simulink model "hcc_sm_v6_circuit2"  (R2024b)
settings: Solver=VariableStepAuto  StartTime=0.0  StopTime=0.2  RelTol=1e-3
libraries: spsSeriesRLCBranchLib x530, spsGtoLib x144, spsDiodeLib x78, spsVoltageMeasurementLib x6, spsGroundLib x2, spsDCVoltageSourceLib x1, spsNonlinearResistorLib x1, spsThreePhaseTransformerTwoWindingsLib x1, spsThreePhaseSourceLib x1, spspowerguiLib x1
(part 2 of 3)

== system hcc_sm_v6_circuit2/Bridge4/Segment3 ==
  gate : Inport
  C{101..106} (6 alike) : spsSeriesRLCBranchLib/Series RLC Branch  LConnTagsString=__new0  RConnTagsString=__new0  BranchType=C  Resistance=350  Inductance=107.42e-03  SetiL0=off  InitialCurrent=0  Capacitance=2.2*1e-6  Setx0=off  InitialVoltage=0  Measurements=None
  Gto{1..6} (6 alike) : spsGtoLib/Gto  Ron=0.226e-6  Lon=0  Vf=1.2  Tf=10e-6  Tt=20e-6  IC=0  Rs=161.25e3  Cs=0  Measurements=off
  R{101..106} (6 alike) : spsSeriesRLCBranchLib/Series RLC Branch  LConnTagsString=__new0  RConnTagsString=__new0  BranchType=R  Resistance=36  Inductance=107.42e-03  SetiL0=off  InitialCurrent=0  Capacitance=2.62e-06  Setx0=off  InitialVoltage=0  Measurements=None
  R{201..206} (6 alike) : spsSeriesRLCBranchLib/Series RLC Branch  LConnTagsString=__new0  RConnTagsString=__new0  BranchType=R  Resistance=88  Inductance=107.42e-03  SetiL0=off  InitialCurrent=0  Capacitance=2.62e-06  Setx0=off  InitialVoltage=0  Measurements=None
  R301_replace : spsDiodeLib/Diode  Ron=0.2624  Lon=0  Vf=11825.10104  IC=0  UseSnubber=0  Rs=1e6  Cs=0  Measurements=on
  R301_replace1 : spsDiodeLib/Diode  Ron=0.2624  Lon=0  Vf=11825.10104  IC=0  UseSnubber=0  Rs=1e6  Cs=0  Measurements=on
  R301_replace2 : spsDiodeLib/Diode  Ron=0.2624  Lon=0  Vf=11825.10104  IC=0  UseSnubber=0  Rs=1e6  Cs=0  Measurements=on
  SaturableReactor : Subsystem
  top : PMIOPort  Side=Left
  bottom : PMIOPort  Port=2  Side=Right
  wires:
  gate/1 -> Gto1/1, Gto2/1, Gto5/1, Gto6/1, Gto4/1, Gto3/1
  connections:
  R106/RConn1 -- C106/LConn1
  R105/RConn1 -- C105/LConn1
  R104/RConn1 -- C104/LConn1
  R103/RConn1 -- C103/LConn1
  C102/LConn1 -- R102/RConn1
  C101/LConn1 -- R101/RConn1
  SaturableReactor/LConn1 -- top/RConn1
  bottom/RConn1 -- R206/RConn1 -- Gto6/RConn1 -- C106/RConn1 -- R301_replace2/RConn1
  R301_replace2/LConn1 -- R301_replace1/RConn1 -- R204/RConn1 -- R205/LConn1 -- Gto4/RConn1 -- Gto5/LConn1 -- C104/RConn1 -- R105/LConn1
  R301_replace1/LConn1 -- R301_replace/RConn1 -- R202/RConn1 -- R103/LConn1 -- Gto2/RConn1 -- Gto3/LConn1 -- C102/RConn1 -- R203/LConn1
  R206/LConn1 -- Gto5/RConn1 -- Gto6/LConn1 -- R106/LConn1 -- C105/RConn1 -- R205/RConn1
  R301_replace/LConn1 -- R101/LConn1 -- SaturableReactor/RConn1 -- Gto1/LConn1 -- R201/LConn1
  R104/LConn1 -- Gto3/RConn1 -- Gto4/LConn1 -- C103/RConn1 -- R204/LConn1 -- R203/RConn1
  R202/LConn1 -- R102/LConn1 -- C101/RConn1 -- Gto1/RConn1 -- Gto2/LConn1 -- R201/RConn1

== system hcc_sm_v6_circuit2/Bridge4/Segment4 ==
  gate : Inport
  C{101..106} (6 alike) : spsSeriesRLCBranchLib/Series RLC Branch  LConnTagsString=__new0  RConnTagsString=__new0  BranchType=C  Resistance=350  Inductance=107.42e-03  SetiL0=off  InitialCurrent=0  Capacitance=2.2*1e-6  Setx0=off  InitialVoltage=0  Measurements=None
  Gto{1..6} (6 alike) : spsGtoLib/Gto  Ron=0.226e-6  Lon=0  Vf=1.2  Tf=10e-6  Tt=20e-6  IC=0  Rs=161.25e3  Cs=0  Measurements=off
  R{101..106} (6 alike) : spsSeriesRLCBranchLib/Series RLC Branch  LConnTagsString=__new0  RConnTagsString=__new0  BranchType=R  Resistance=36  Inductance=107.42e-03  SetiL0=off  InitialCurrent=0  Capacitance=2.62e-06  Setx0=off  InitialVoltage=0  Measurements=None
  R{201..206} (6 alike) : spsSeriesRLCBranchLib/Series RLC Branch  LConnTagsString=__new0  RConnTagsString=__new0  BranchType=R  Resistance=88  Inductance=107.42e-03  SetiL0=off  InitialCurrent=0  Capacitance=2.62e-06  Setx0=off  InitialVoltage=0  Measurements=None
  R301_replace : spsDiodeLib/Diode  Ron=0.2624  Lon=0  Vf=11825.10104  IC=0  UseSnubber=0  Rs=1e6  Cs=0  Measurements=on
  R301_replace1 : spsDiodeLib/Diode  Ron=0.2624  Lon=0  Vf=11825.10104  IC=0  UseSnubber=0  Rs=1e6  Cs=0  Measurements=on
  R301_replace2 : spsDiodeLib/Diode  Ron=0.2624  Lon=0  Vf=11825.10104  IC=0  UseSnubber=0  Rs=1e6  Cs=0  Measurements=on
  SaturableReactor : Subsystem
  top : PMIOPort  Side=Left
  bottom : PMIOPort  Port=2  Side=Right
  wires:
  gate/1 -> Gto3/1, Gto4/1, Gto6/1, Gto5/1, Gto2/1, Gto1/1
  connections:
  R201/RConn1 -- Gto2/LConn1 -- Gto1/RConn1 -- C101/RConn1 -- R102/LConn1 -- R202/LConn1
  R203/RConn1 -- R204/LConn1 -- C103/RConn1 -- Gto4/LConn1 -- Gto3/RConn1 -- R104/LConn1
  R201/LConn1 -- Gto1/LConn1 -- SaturableReactor/RConn1 -- R101/LConn1 -- R301_replace/LConn1
  R205/RConn1 -- C105/RConn1 -- R106/LConn1 -- Gto6/LConn1 -- Gto5/RConn1 -- R206/LConn1
  R203/LConn1 -- C102/RConn1 -- Gto3/LConn1 -- Gto2/RConn1 -- R103/LConn1 -- R202/RConn1 -- R301_replace/RConn1 -- R301_replace1/LConn1
  R105/LConn1 -- C104/RConn1 -- Gto5/LConn1 -- Gto4/RConn1 -- R205/LConn1 -- R204/RConn1 -- R301_replace1/RConn1 -- R301_replace2/LConn1
  R301_replace2/RConn1 -- C106/RConn1 -- Gto6/RConn1 -- R206/RConn1 -- bottom/RConn1
  SaturableReactor/LConn1 -- top/RConn1
  C101/LConn1 -- R101/RConn1
  C102/LConn1 -- R102/RConn1
  R103/RConn1 -- C103/LConn1
  R104/RConn1 -- C104/LConn1
  R105/RConn1 -- C105/LConn1
  R106/RConn1 -- C106/LConn1

== system hcc_sm_v6_circuit2/Bridge5/Segment1 ==
  gate : Inport
  C{101..106} (6 alike) : spsSeriesRLCBranchLib/Series RLC Branch  LConnTagsString=__new0  RConnTagsString=__new0  BranchType=C  Resistance=350  Inductance=107.42e-03  SetiL0=off  InitialCurrent=0  Capacitance=2.2*1e-6  Setx0=off  InitialVoltage=0  Measurements=None
  Gto{1..6} (6 alike) : spsGtoLib/Gto  Ron=0.226e-6  Lon=0  Vf=1.2  Tf=10e-6  Tt=20e-6  IC=0  Rs=161.25e3  Cs=0  Measurements=off
  R{101..106} (6 alike) : spsSeriesRLCBranchLib/Series RLC Branch  LConnTagsString=__new0  RConnTagsString=__new0  BranchType=R  Resistance=36  Inductance=107.42e-03  SetiL0=off  InitialCurrent=0  Capacitance=2.62e-06  Setx0=off  InitialVoltage=0  Measurements=None
  R{201..206} (6 alike) : spsSeriesRLCBranchLib/Series RLC Branch  LConnTagsString=__new0  RConnTagsString=__new0  BranchType=R  Resistance=88  Inductance=107.42e-03  SetiL0=off  InitialCurrent=0  Capacitance=2.62e-06  Setx0=off  InitialVoltage=0  Measurements=None
  R301_replace : spsDiodeLib/Diode  Ron=0.2624  Lon=0  Vf=11825.10104  IC=0  UseSnubber=0  Rs=1e6  Cs=0  Measurements=on
  R301_replace1 : spsDiodeLib/Diode  Ron=0.2624  Lon=0  Vf=11825.10104  IC=0  UseSnubber=0  Rs=1e6  Cs=0  Measurements=on
  R301_replace2 : spsDiodeLib/Diode  Ron=0.2624  Lon=0  Vf=11825.10104  IC=0  UseSnubber=0  Rs=1e6  Cs=0  Measurements=on
  SaturableReactor : Subsystem
  top : PMIOPort  Side=Left
  bottom : PMIOPort  Port=2  Side=Right
  wires:
  gate/1 -> Gto3/1, Gto4/1, Gto6/1, Gto5/1, Gto2/1, Gto1/1
  connections:
  R201/RConn1 -- Gto2/LConn1 -- Gto1/RConn1 -- C101/RConn1 -- R102/LConn1 -- R202/LConn1
  R203/RConn1 -- R204/LConn1 -- C103/RConn1 -- Gto4/LConn1 -- Gto3/RConn1 -- R104/LConn1
  R201/LConn1 -- Gto1/LConn1 -- SaturableReactor/RConn1 -- R101/LConn1 -- R301_replace/LConn1
  R205/RConn1 -- C105/RConn1 -- R106/LConn1 -- Gto6/LConn1 -- Gto5/RConn1 -- R206/LConn1
  R203/LConn1 -- C102/RConn1 -- Gto3/LConn1 -- Gto2/RConn1 -- R103/LConn1 -- R202/RConn1 -- R301_replace/RConn1 -- R301_replace1/LConn1
  R105/LConn1 -- C104/RConn1 -- Gto5/LConn1 -- Gto4/RConn1 -- R205/LConn1 -- R204/RConn1 -- R301_replace1/RConn1 -- R301_replace2/LConn1
  R301_replace2/RConn1 -- C106/RConn1 -- Gto6/RConn1 -- R206/RConn1 -- bottom/RConn1
  SaturableReactor/LConn1 -- top/RConn1
  C101/LConn1 -- R101/RConn1
  C102/LConn1 -- R102/RConn1
  R103/RConn1 -- C103/LConn1
  R104/RConn1 -- C104/LConn1
  R105/RConn1 -- C105/LConn1
  R106/RConn1 -- C106/LConn1

== system hcc_sm_v6_circuit2/Bridge5/Segment2 ==
  gate : Inport
  C{101..106} (6 alike) : spsSeriesRLCBranchLib/Series RLC Branch  LConnTagsString=__new0  RConnTagsString=__new0  BranchType=C  Resistance=350  Inductance=107.42e-03  SetiL0=off  InitialCurrent=0  Capacitance=2.2*1e-6  Setx0=off  InitialVoltage=0  Measurements=None
  Gto{1..6} (6 alike) : spsGtoLib/Gto  Ron=0.226e-6  Lon=0  Vf=1.2  Tf=10e-6  Tt=20e-6  IC=0  Rs=161.25e3  Cs=0  Measurements=off
  R{101..106} (6 alike) : spsSeriesRLCBranchLib/Series RLC Branch  LConnTagsString=__new0  RConnTagsString=__new0  BranchType=R  Resistance=36  Inductance=107.42e-03  SetiL0=off  InitialCurrent=0  Capacitance=2.62e-06  Setx0=off  InitialVoltage=0  Measurements=None
  R{201..206} (6 alike) : spsSeriesRLCBranchLib/Series RLC Branch  LConnTagsString=__new0  RConnTagsString=__new0  BranchType=R  Resistance=88  Inductance=107.42e-03  SetiL0=off  InitialCurrent=0  Capacitance=2.62e-06  Setx0=off  InitialVoltage=0  Measurements=None
  R301_replace : spsDiodeLib/Diode  Ron=0.2624  Lon=0  Vf=11825.10104  IC=0  UseSnubber=0  Rs=1e6  Cs=0  Measurements=on
  R301_replace1 : spsDiodeLib/Diode  Ron=0.2624  Lon=0  Vf=11825.10104  IC=0  UseSnubber=0  Rs=1e6  Cs=0  Measurements=on
  R301_replace2 : spsDiodeLib/Diode  Ron=0.2624  Lon=0  Vf=11825.10104  IC=0  UseSnubber=0  Rs=1e6  Cs=0  Measurements=on
  SaturableReactor : Subsystem
  top : PMIOPort  Side=Left
  bottom : PMIOPort  Port=2  Side=Right
  wires:
  gate/1 -> Gto1/1, Gto2/1, Gto5/1, Gto6/1, Gto4/1, Gto3/1
  connections:
  R106/RConn1 -- C106/LConn1
  R105/RConn1 -- C105/LConn1
  R104/RConn1 -- C104/LConn1
  R103/RConn1 -- C103/LConn1
  C102/LConn1 -- R102/RConn1
  C101/LConn1 -- R101/RConn1
  SaturableReactor/LConn1 -- top/RConn1
  bottom/RConn1 -- R206/RConn1 -- Gto6/RConn1 -- C106/RConn1 -- R301_replace2/RConn1
  R301_replace2/LConn1 -- R301_replace1/RConn1 -- R204/RConn1 -- R205/LConn1 -- Gto4/RConn1 -- Gto5/LConn1 -- C104/RConn1 -- R105/LConn1
  R301_replace1/LConn1 -- R301_replace/RConn1 -- R202/RConn1 -- R103/LConn1 -- Gto2/RConn1 -- Gto3/LConn1 -- C102/RConn1 -- R203/LConn1
  R206/LConn1 -- Gto5/RConn1 -- Gto6/LConn1 -- R106/LConn1 -- C105/RConn1 -- R205/RConn1
  R301_replace/LConn1 -- R101/LConn1 -- SaturableReactor/RConn1 -- Gto1/LConn1 -- R201/LConn1
  R104/LConn1 -- Gto3/RConn1 -- Gto4/LConn1 -- C103/RConn1 -- R204/LConn1 -- R203/RConn1
  R202/LConn1 -- R102/LConn1 -- C101/RConn1 -- Gto1/RConn1 -- Gto2/LConn1 -- R201/RConn1

== system hcc_sm_v6_circuit2/Bridge5/Segment3 ==
  gate : Inport
  C{101..106} (6 alike) : spsSeriesRLCBranchLib/Series RLC Branch  LConnTagsString=__new0  RConnTagsString=__new0  BranchType=C  Resistance=350  Inductance=107.42e-03  SetiL0=off  InitialCurrent=0  Capacitance=2.2*1e-6  Setx0=off  InitialVoltage=0  Measurements=None
  Gto{1..6} (6 alike) : spsGtoLib/Gto  Ron=0.226e-6  Lon=0  Vf=1.2  Tf=10e-6  Tt=20e-6  IC=0  Rs=161.25e3  Cs=0  Measurements=off
  R{101..106} (6 alike) : spsSeriesRLCBranchLib/Series RLC Branch  LConnTagsString=__new0  RConnTagsString=__new0  BranchType=R  Resistance=36  Inductance=107.42e-03  SetiL0=off  InitialCurrent=0  Capacitance=2.62e-06  Setx0=off  InitialVoltage=0  Measurements=None
  R{201..206} (6 alike) : spsSeriesRLCBranchLib/Series RLC Branch  LConnTagsString=__new0  RConnTagsString=__new0  BranchType=R  Resistance=88  Inductance=107.42e-03  SetiL0=off  InitialCurrent=0  Capacitance=2.62e-06  Setx0=off  InitialVoltage=0  Measurements=None
  R301_replace : spsDiodeLib/Diode  Ron=0.2624  Lon=0  Vf=11825.10104  IC=0  UseSnubber=0  Rs=1e6  Cs=0  Measurements=on
  R301_replace1 : spsDiodeLib/Diode  Ron=0.2624  Lon=0  Vf=11825.10104  IC=0  UseSnubber=0  Rs=1e6  Cs=0  Measurements=on
  R301_replace2 : spsDiodeLib/Diode  Ron=0.2624  Lon=0  Vf=11825.10104  IC=0  UseSnubber=0  Rs=1e6  Cs=0  Measurements=on
  SaturableReactor : Subsystem
  top : PMIOPort  Side=Left
  bottom : PMIOPort  Port=2  Side=Right
  wires:
  gate/1 -> Gto3/1, Gto4/1, Gto6/1, Gto5/1, Gto2/1, Gto1/1
  connections:
  R201/RConn1 -- Gto2/LConn1 -- Gto1/RConn1 -- C101/RConn1 -- R102/LConn1 -- R202/LConn1
  R203/RConn1 -- R204/LConn1 -- C103/RConn1 -- Gto4/LConn1 -- Gto3/RConn1 -- R104/LConn1
  R201/LConn1 -- Gto1/LConn1 -- SaturableReactor/RConn1 -- R101/LConn1 -- R301_replace/LConn1
  R205/RConn1 -- C105/RConn1 -- R106/LConn1 -- Gto6/LConn1 -- Gto5/RConn1 -- R206/LConn1
  R203/LConn1 -- C102/RConn1 -- Gto3/LConn1 -- Gto2/RConn1 -- R103/LConn1 -- R202/RConn1 -- R301_replace/RConn1 -- R301_replace1/LConn1
  R105/LConn1 -- C104/RConn1 -- Gto5/LConn1 -- Gto4/RConn1 -- R205/LConn1 -- R204/RConn1 -- R301_replace1/RConn1 -- R301_replace2/LConn1
  R301_replace2/RConn1 -- C106/RConn1 -- Gto6/RConn1 -- R206/RConn1 -- bottom/RConn1
  SaturableReactor/LConn1 -- top/RConn1
  C101/LConn1 -- R101/RConn1
  C102/LConn1 -- R102/RConn1
  R103/RConn1 -- C103/LConn1
  R104/RConn1 -- C104/LConn1
  R105/RConn1 -- C105/LConn1
  R106/RConn1 -- C106/LConn1

== system hcc_sm_v6_circuit2/Bridge5/Segment4 ==
  gate : Inport
  C{101..106} (6 alike) : spsSeriesRLCBranchLib/Series RLC Branch  LConnTagsString=__new0  RConnTagsString=__new0  BranchType=C  Resistance=350  Inductance=107.42e-03  SetiL0=off  InitialCurrent=0  Capacitance=2.2*1e-6  Setx0=off  InitialVoltage=0  Measurements=None
  Gto{1..6} (6 alike) : spsGtoLib/Gto  Ron=0.226e-6  Lon=0  Vf=1.2  Tf=10e-6  Tt=20e-6  IC=0  Rs=161.25e3  Cs=0  Measurements=off
  R{101..106} (6 alike) : spsSeriesRLCBranchLib/Series RLC Branch  LConnTagsString=__new0  RConnTagsString=__new0  BranchType=R  Resistance=36  Inductance=107.42e-03  SetiL0=off  InitialCurrent=0  Capacitance=2.62e-06  Setx0=off  InitialVoltage=0  Measurements=None
  R{201..206} (6 alike) : spsSeriesRLCBranchLib/Series RLC Branch  LConnTagsString=__new0  RConnTagsString=__new0  BranchType=R  Resistance=88  Inductance=107.42e-03  SetiL0=off  InitialCurrent=0  Capacitance=2.62e-06  Setx0=off  InitialVoltage=0  Measurements=None
  R301_replace : spsDiodeLib/Diode  Ron=0.2624  Lon=0  Vf=11825.10104  IC=0  UseSnubber=0  Rs=1e6  Cs=0  Measurements=on
  R301_replace1 : spsDiodeLib/Diode  Ron=0.2624  Lon=0  Vf=11825.10104  IC=0  UseSnubber=0  Rs=1e6  Cs=0  Measurements=on
  R301_replace2 : spsDiodeLib/Diode  Ron=0.2624  Lon=0  Vf=11825.10104  IC=0  UseSnubber=0  Rs=1e6  Cs=0  Measurements=on
  SaturableReactor : Subsystem
  top : PMIOPort  Side=Left
  bottom : PMIOPort  Port=2  Side=Right
  wires:
  gate/1 -> Gto1/1, Gto2/1, Gto5/1, Gto6/1, Gto4/1, Gto3/1
  connections:
  R106/RConn1 -- C106/LConn1
  R105/RConn1 -- C105/LConn1
  R104/RConn1 -- C104/LConn1
  R103/RConn1 -- C103/LConn1
  C102/LConn1 -- R102/RConn1
  C101/LConn1 -- R101/RConn1
  SaturableReactor/LConn1 -- top/RConn1
  bottom/RConn1 -- R206/RConn1 -- Gto6/RConn1 -- C106/RConn1 -- R301_replace2/RConn1
  R301_replace2/LConn1 -- R301_replace1/RConn1 -- R204/RConn1 -- R205/LConn1 -- Gto4/RConn1 -- Gto5/LConn1 -- C104/RConn1 -- R105/LConn1
  R301_replace1/LConn1 -- R301_replace/RConn1 -- R202/RConn1 -- R103/LConn1 -- Gto2/RConn1 -- Gto3/LConn1 -- C102/RConn1 -- R203/LConn1
  R206/LConn1 -- Gto5/RConn1 -- Gto6/LConn1 -- R106/LConn1 -- C105/RConn1 -- R205/RConn1
  R301_replace/LConn1 -- R101/LConn1 -- SaturableReactor/RConn1 -- Gto1/LConn1 -- R201/LConn1
  R104/LConn1 -- Gto3/RConn1 -- Gto4/LConn1 -- C103/RConn1 -- R204/LConn1 -- R203/RConn1
  R202/LConn1 -- R102/LConn1 -- C101/RConn1 -- Gto1/RConn1 -- Gto2/LConn1 -- R201/RConn1

== system hcc_sm_v6_circuit2/Bridge6/Segment1 ==
  gate : Inport
  C{101..106} (6 alike) : spsSeriesRLCBranchLib/Series RLC Branch  LConnTagsString=__new0  RConnTagsString=__new0  BranchType=C  Resistance=350  Inductance=107.42e-03  SetiL0=off  InitialCurrent=0  Capacitance=2.2*1e-6  Setx0=off  InitialVoltage=0  Measurements=None
  Gto{1..6} (6 alike) : spsGtoLib/Gto  Ron=0.226e-6  Lon=0  Vf=1.2  Tf=10e-6  Tt=20e-6  IC=0  Rs=161.25e3  Cs=0  Measurements=off
  R{101..106} (6 alike) : spsSeriesRLCBranchLib/Series RLC Branch  LConnTagsString=__new0  RConnTagsString=__new0  BranchType=R  Resistance=36  Inductance=107.42e-03  SetiL0=off  InitialCurrent=0  Capacitance=2.62e-06  Setx0=off  InitialVoltage=0  Measurements=None
  R{201..206} (6 alike) : spsSeriesRLCBranchLib/Series RLC Branch  LConnTagsString=__new0  RConnTagsString=__new0  BranchType=R  Resistance=88  Inductance=107.42e-03  SetiL0=off  InitialCurrent=0  Capacitance=2.62e-06  Setx0=off  InitialVoltage=0  Measurements=None
  R301_replace : spsDiodeLib/Diode  Ron=0.2624  Lon=0  Vf=11825.10104  IC=0  UseSnubber=0  Rs=1e6  Cs=0  Measurements=on
  R301_replace1 : spsDiodeLib/Diode  Ron=0.2624  Lon=0  Vf=11825.10104  IC=0  UseSnubber=0  Rs=1e6  Cs=0  Measurements=on
  R301_replace2 : spsDiodeLib/Diode  Ron=0.2624  Lon=0  Vf=11825.10104  IC=0  UseSnubber=0  Rs=1e6  Cs=0  Measurements=on
  SaturableReactor : Subsystem
  top : PMIOPort  Side=Left
  bottom : PMIOPort  Port=2  Side=Right
  wires:
  gate/1 -> Gto3/1, Gto4/1, Gto6/1, Gto5/1, Gto2/1, Gto1/1
  connections:
  R201/RConn1 -- Gto2/LConn1 -- Gto1/RConn1 -- C101/RConn1 -- R102/LConn1 -- R202/LConn1
  R203/RConn1 -- R204/LConn1 -- C103/RConn1 -- Gto4/LConn1 -- Gto3/RConn1 -- R104/LConn1
  R201/LConn1 -- Gto1/LConn1 -- SaturableReactor/RConn1 -- R101/LConn1 -- R301_replace/LConn1
  R205/RConn1 -- C105/RConn1 -- R106/LConn1 -- Gto6/LConn1 -- Gto5/RConn1 -- R206/LConn1
  R203/LConn1 -- C102/RConn1 -- Gto3/LConn1 -- Gto2/RConn1 -- R103/LConn1 -- R202/RConn1 -- R301_replace/RConn1 -- R301_replace1/LConn1
  R105/LConn1 -- C104/RConn1 -- Gto5/LConn1 -- Gto4/RConn1 -- R205/LConn1 -- R204/RConn1 -- R301_replace1/RConn1 -- R301_replace2/LConn1
  R301_replace2/RConn1 -- C106/RConn1 -- Gto6/RConn1 -- R206/RConn1 -- bottom/RConn1
  SaturableReactor/LConn1 -- top/RConn1
  C101/LConn1 -- R101/RConn1
  C102/LConn1 -- R102/RConn1
  R103/RConn1 -- C103/LConn1
  R104/RConn1 -- C104/LConn1
  R105/RConn1 -- C105/LConn1
  R106/RConn1 -- C106/LConn1

== system hcc_sm_v6_circuit2/Bridge6/Segment2 ==
  gate : Inport
  C{101..106} (6 alike) : spsSeriesRLCBranchLib/Series RLC Branch  LConnTagsString=__new0  RConnTagsString=__new0  BranchType=C  Resistance=350  Inductance=107.42e-03  SetiL0=off  InitialCurrent=0  Capacitance=2.2*1e-6  Setx0=off  InitialVoltage=0  Measurements=None
  Gto{1..6} (6 alike) : spsGtoLib/Gto  Ron=0.226e-6  Lon=0  Vf=1.2  Tf=10e-6  Tt=20e-6  IC=0  Rs=161.25e3  Cs=0  Measurements=off
  R{101..106} (6 alike) : spsSeriesRLCBranchLib/Series RLC Branch  LConnTagsString=__new0  RConnTagsString=__new0  BranchType=R  Resistance=36  Inductance=107.42e-03  SetiL0=off  InitialCurrent=0  Capacitance=2.62e-06  Setx0=off  InitialVoltage=0  Measurements=None
  R{201..206} (6 alike) : spsSeriesRLCBranchLib/Series RLC Branch  LConnTagsString=__new0  RConnTagsString=__new0  BranchType=R  Resistance=88  Inductance=107.42e-03  SetiL0=off  InitialCurrent=0  Capacitance=2.62e-06  Setx0=off  InitialVoltage=0  Measurements=None
  R301_replace : spsDiodeLib/Diode  Ron=0.2624  Lon=0  Vf=11825.10104  IC=0  UseSnubber=0  Rs=1e6  Cs=0  Measurements=on
  R301_replace1 : spsDiodeLib/Diode  Ron=0.2624  Lon=0  Vf=11825.10104  IC=0  UseSnubber=0  Rs=1e6  Cs=0  Measurements=on
  R301_replace2 : spsDiodeLib/Diode  Ron=0.2624  Lon=0  Vf=11825.10104  IC=0  UseSnubber=0  Rs=1e6  Cs=0  Measurements=on
  SaturableReactor : Subsystem
  top : PMIOPort  Side=Left
  bottom : PMIOPort  Port=2  Side=Right
  wires:
  gate/1 -> Gto1/1, Gto2/1, Gto5/1, Gto6/1, Gto4/1, Gto3/1
  connections:
  R106/RConn1 -- C106/LConn1
  R105/RConn1 -- C105/LConn1
  R104/RConn1 -- C104/LConn1
  R103/RConn1 -- C103/LConn1
  C102/LConn1 -- R102/RConn1
  C101/LConn1 -- R101/RConn1
  SaturableReactor/LConn1 -- top/RConn1
  bottom/RConn1 -- R206/RConn1 -- Gto6/RConn1 -- C106/RConn1 -- R301_replace2/RConn1
  R301_replace2/LConn1 -- R301_replace1/RConn1 -- R204/RConn1 -- R205/LConn1 -- Gto4/RConn1 -- Gto5/LConn1 -- C104/RConn1 -- R105/LConn1
  R301_replace1/LConn1 -- R301_replace/RConn1 -- R202/RConn1 -- R103/LConn1 -- Gto2/RConn1 -- Gto3/LConn1 -- C102/RConn1 -- R203/LConn1
  R206/LConn1 -- Gto5/RConn1 -- Gto6/LConn1 -- R106/LConn1 -- C105/RConn1 -- R205/RConn1
  R301_replace/LConn1 -- R101/LConn1 -- SaturableReactor/RConn1 -- Gto1/LConn1 -- R201/LConn1
  R104/LConn1 -- Gto3/RConn1 -- Gto4/LConn1 -- C103/RConn1 -- R204/LConn1 -- R203/RConn1
  R202/LConn1 -- R102/LConn1 -- C101/RConn1 -- Gto1/RConn1 -- Gto2/LConn1 -- R201/RConn1

== system hcc_sm_v6_circuit2/Bridge6/Segment3 ==
  gate : Inport
  C{101..106} (6 alike) : spsSeriesRLCBranchLib/Series RLC Branch  LConnTagsString=__new0  RConnTagsString=__new0  BranchType=C  Resistance=350  Inductance=107.42e-03  SetiL0=off  InitialCurrent=0  Capacitance=2.2*1e-6  Setx0=off  InitialVoltage=0  Measurements=None
  Gto{1..6} (6 alike) : spsGtoLib/Gto  Ron=0.226e-6  Lon=0  Vf=1.2  Tf=10e-6  Tt=20e-6  IC=0  Rs=161.25e3  Cs=0  Measurements=off
  R{101..106} (6 alike) : spsSeriesRLCBranchLib/Series RLC Branch  LConnTagsString=__new0  RConnTagsString=__new0  BranchType=R  Resistance=36  Inductance=107.42e-03  SetiL0=off  InitialCurrent=0  Capacitance=2.62e-06  Setx0=off  InitialVoltage=0  Measurements=None
  R{201..206} (6 alike) : spsSeriesRLCBranchLib/Series RLC Branch  LConnTagsString=__new0  RConnTagsString=__new0  BranchType=R  Resistance=88  Inductance=107.42e-03  SetiL0=off  InitialCurrent=0  Capacitance=2.62e-06  Setx0=off  InitialVoltage=0  Measurements=None
  R301_replace : spsDiodeLib/Diode  Ron=0.2624  Lon=0  Vf=11825.10104  IC=0  UseSnubber=0  Rs=1e6  Cs=0  Measurements=on
  R301_replace1 : spsDiodeLib/Diode  Ron=0.2624  Lon=0  Vf=11825.10104  IC=0  UseSnubber=0  Rs=1e6  Cs=0  Measurements=on
  R301_replace2 : spsDiodeLib/Diode  Ron=0.2624  Lon=0  Vf=11825.10104  IC=0  UseSnubber=0  Rs=1e6  Cs=0  Measurements=on
  SaturableReactor : Subsystem
  top : PMIOPort  Side=Left
  bottom : PMIOPort  Port=2  Side=Right
  wires:
  gate/1 -> Gto3/1, Gto4/1, Gto6/1, Gto5/1, Gto2/1, Gto1/1
  connections:
  R201/RConn1 -- Gto2/LConn1 -- Gto1/RConn1 -- C101/RConn1 -- R102/LConn1 -- R202/LConn1
  R203/RConn1 -- R204/LConn1 -- C103/RConn1 -- Gto4/LConn1 -- Gto3/RConn1 -- R104/LConn1
  R201/LConn1 -- Gto1/LConn1 -- SaturableReactor/RConn1 -- R101/LConn1 -- R301_replace/LConn1
  R205/RConn1 -- C105/RConn1 -- R106/LConn1 -- Gto6/LConn1 -- Gto5/RConn1 -- R206/LConn1
  R203/LConn1 -- C102/RConn1 -- Gto3/LConn1 -- Gto2/RConn1 -- R103/LConn1 -- R202/RConn1 -- R301_replace/RConn1 -- R301_replace1/LConn1
  R105/LConn1 -- C104/RConn1 -- Gto5/LConn1 -- Gto4/RConn1 -- R205/LConn1 -- R204/RConn1 -- R301_replace1/RConn1 -- R301_replace2/LConn1
  R301_replace2/RConn1 -- C106/RConn1 -- Gto6/RConn1 -- R206/RConn1 -- bottom/RConn1
  SaturableReactor/LConn1 -- top/RConn1
  C101/LConn1 -- R101/RConn1
  C102/LConn1 -- R102/RConn1
  R103/RConn1 -- C103/LConn1
  R104/RConn1 -- C104/LConn1
  R105/RConn1 -- C105/LConn1
  R106/RConn1 -- C106/LConn1

== system hcc_sm_v6_circuit2/Bridge6/Segment4 ==
  gate : Inport
  C{101..106} (6 alike) : spsSeriesRLCBranchLib/Series RLC Branch  LConnTagsString=__new0  RConnTagsString=__new0  BranchType=C  Resistance=350  Inductance=107.42e-03  SetiL0=off  InitialCurrent=0  Capacitance=2.2*1e-6  Setx0=off  InitialVoltage=0  Measurements=None
  Gto{1..6} (6 alike) : spsGtoLib/Gto  Ron=0.226e-6  Lon=0  Vf=1.2  Tf=10e-6  Tt=20e-6  IC=0  Rs=161.25e3  Cs=0  Measurements=off
  R{101..106} (6 alike) : spsSeriesRLCBranchLib/Series RLC Branch  LConnTagsString=__new0  RConnTagsString=__new0  BranchType=R  Resistance=36  Inductance=107.42e-03  SetiL0=off  InitialCurrent=0  Capacitance=2.62e-06  Setx0=off  InitialVoltage=0  Measurements=None
  R{201..206} (6 alike) : spsSeriesRLCBranchLib/Series RLC Branch  LConnTagsString=__new0  RConnTagsString=__new0  BranchType=R  Resistance=88  Inductance=107.42e-03  SetiL0=off  InitialCurrent=0  Capacitance=2.62e-06  Setx0=off  InitialVoltage=0  Measurements=None
  R301_replace : spsDiodeLib/Diode  Ron=0.2624  Lon=0  Vf=11825.10104  IC=0  UseSnubber=0  Rs=1e6  Cs=0  Measurements=on
  R301_replace1 : spsDiodeLib/Diode  Ron=0.2624  Lon=0  Vf=11825.10104  IC=0  UseSnubber=0  Rs=1e6  Cs=0  Measurements=on
  R301_replace2 : spsDiodeLib/Diode  Ron=0.2624  Lon=0  Vf=11825.10104  IC=0  UseSnubber=0  Rs=1e6  Cs=0  Measurements=on
  SaturableReactor : Subsystem
  top : PMIOPort  Side=Left
  bottom : PMIOPort  Port=2  Side=Right
  wires:
  gate/1 -> Gto1/1, Gto2/1, Gto5/1, Gto6/1, Gto4/1, Gto3/1
  connections:
  R106/RConn1 -- C106/LConn1
  R105/RConn1 -- C105/LConn1
  R104/RConn1 -- C104/LConn1
  R103/RConn1 -- C103/LConn1
  C102/LConn1 -- R102/RConn1
  C101/LConn1 -- R101/RConn1
  SaturableReactor/LConn1 -- top/RConn1
  bottom/RConn1 -- R206/RConn1 -- Gto6/RConn1 -- C106/RConn1 -- R301_replace2/RConn1
  R301_replace2/LConn1 -- R301_replace1/RConn1 -- R204/RConn1 -- R205/LConn1 -- Gto4/RConn1 -- Gto5/LConn1 -- C104/RConn1 -- R105/LConn1
  R301_replace1/LConn1 -- R301_replace/RConn1 -- R202/RConn1 -- R103/LConn1 -- Gto2/RConn1 -- Gto3/LConn1 -- C102/RConn1 -- R203/LConn1
  R206/LConn1 -- Gto5/RConn1 -- Gto6/LConn1 -- R106/LConn1 -- C105/RConn1 -- R205/RConn1
  R301_replace/LConn1 -- R101/LConn1 -- SaturableReactor/RConn1 -- Gto1/LConn1 -- R201/LConn1
  R104/LConn1 -- Gto3/RConn1 -- Gto4/LConn1 -- C103/RConn1 -- R204/LConn1 -- R203/RConn1
  R202/LConn1 -- R102/LConn1 -- C101/RConn1 -- Gto1/RConn1 -- Gto2/LConn1 -- R201/RConn1

== system hcc_sm_v6_circuit2/Bridge1/Segment1/SaturableReactor ==
  note: C
  Cs : spsSeriesRLCBranchLib/Series RLC Branch  LConnTagsString=__new0  RConnTagsString=__new0  BranchType=C  Resistance=88  Inductance=6.3e-6  SetiL0=off  InitialCurrent=0  Capacitance=250e-12  Setx0=off  InitialVoltage=0  Measurements=None
  LAir : spsSeriesRLCBranchLib/Series RLC Branch  LConnTagsString=__new0  RConnTagsString=__new0  BranchType=L  Resistance=88  Inductance=6.3e-6  SetiL0=off  InitialCurrent=0  Capacitance=2.62e-06  Setx0=off  InitialVoltage=0  Measurements=None
  Lm : spsSeriesRLCBranchLib/Series RLC Branch  LConnTagsString=__new0  RConnTagsString=__new0  BranchType=L  Resistance=88  Inductance=524.8e-6  SetiL0=off  InitialCurrent=0  Capacitance=2.62e-06  Setx0=off  InitialVoltage=0  Measurements=None
  Re : spsSeriesRLCBranchLib/Series RLC Branch  LConnTagsString=__new0  RConnTagsString=__new0  BranchType=R  Resistance=250  Inductance=6.3e-6  SetiL0=off  InitialCurrent=0  Capacitance=2.62e-06  Setx0=off  InitialVoltage=0  Measurements=None
  A : PMIOPort  Side=Left
  B : PMIOPort  Port=2  Side=Right
  connections:
  A/RConn1 -- Cs/LConn1 -- LAir/LConn1
  LAir/RConn1 -- Re/LConn1 -- Lm/LConn1
  Cs/RConn1 -- Lm/RConn1 -- Re/RConn1 -- B/RConn1

== system hcc_sm_v6_circuit2/Bridge1/Segment2/SaturableReactor ==
  note: C
  Cs : spsSeriesRLCBranchLib/Series RLC Branch  LConnTagsString=__new0  RConnTagsString=__new0  BranchType=C  Resistance=88  Inductance=6.3e-6  SetiL0=off  InitialCurrent=0  Capacitance=250e-12  Setx0=off  InitialVoltage=0  Measurements=None
  LAir : spsSeriesRLCBranchLib/Series RLC Branch  LConnTagsString=__new0  RConnTagsString=__new0  BranchType=L  Resistance=88  Inductance=6.3e-6  SetiL0=off  InitialCurrent=0  Capacitance=2.62e-06  Setx0=off  InitialVoltage=0  Measurements=None
  Lm : spsSeriesRLCBranchLib/Series RLC Branch  LConnTagsString=__new0  RConnTagsString=__new0  BranchType=L  Resistance=88  Inductance=524.8e-6  SetiL0=off  InitialCurrent=0  Capacitance=2.62e-06  Setx0=off  InitialVoltage=0  Measurements=None
  Re : spsSeriesRLCBranchLib/Series RLC Branch  LConnTagsString=__new0  RConnTagsString=__new0  BranchType=R  Resistance=250  Inductance=6.3e-6  SetiL0=off  InitialCurrent=0  Capacitance=2.62e-06  Setx0=off  InitialVoltage=0  Measurements=None
  A : PMIOPort  Side=Left
  B : PMIOPort  Port=2  Side=Right
  connections:
  B/RConn1 -- Re/RConn1 -- Lm/RConn1 -- Cs/RConn1
  Lm/LConn1 -- Re/LConn1 -- LAir/RConn1
  LAir/LConn1 -- Cs/LConn1 -- A/RConn1

== system hcc_sm_v6_circuit2/Bridge1/Segment3/SaturableReactor ==
  note: C
  Cs : spsSeriesRLCBranchLib/Series RLC Branch  LConnTagsString=__new0  RConnTagsString=__new0  BranchType=C  Resistance=88  Inductance=6.3e-6  SetiL0=off  InitialCurrent=0  Capacitance=250e-12  Setx0=off  InitialVoltage=0  Measurements=None
  LAir : spsSeriesRLCBranchLib/Series RLC Branch  LConnTagsString=__new0  RConnTagsString=__new0  BranchType=L  Resistance=88  Inductance=6.3e-6  SetiL0=off  InitialCurrent=0  Capacitance=2.62e-06  Setx0=off  InitialVoltage=0  Measurements=None
  Lm : spsSeriesRLCBranchLib/Series RLC Branch  LConnTagsString=__new0  RConnTagsString=__new0  BranchType=L  Resistance=88  Inductance=524.8e-6  SetiL0=off  InitialCurrent=0  Capacitance=2.62e-06  Setx0=off  InitialVoltage=0  Measurements=None
  Re : spsSeriesRLCBranchLib/Series RLC Branch  LConnTagsString=__new0  RConnTagsString=__new0  BranchType=R  Resistance=250  Inductance=6.3e-6  SetiL0=off  InitialCurrent=0  Capacitance=2.62e-06  Setx0=off  InitialVoltage=0  Measurements=None
  A : PMIOPort  Side=Left
  B : PMIOPort  Port=2  Side=Right
  connections:
  A/RConn1 -- Cs/LConn1 -- LAir/LConn1
  LAir/RConn1 -- Re/LConn1 -- Lm/LConn1
  Cs/RConn1 -- Lm/RConn1 -- Re/RConn1 -- B/RConn1

== system hcc_sm_v6_circuit2/Bridge1/Segment4/SaturableReactor ==
  note: C
  Cs : spsSeriesRLCBranchLib/Series RLC Branch  LConnTagsString=__new0  RConnTagsString=__new0  BranchType=C  Resistance=88  Inductance=6.3e-6  SetiL0=off  InitialCurrent=0  Capacitance=250e-12  Setx0=off  InitialVoltage=0  Measurements=None
  LAir : spsSeriesRLCBranchLib/Series RLC Branch  LConnTagsString=__new0  RConnTagsString=__new0  BranchType=L  Resistance=88  Inductance=6.3e-6  SetiL0=off  InitialCurrent=0  Capacitance=2.62e-06  Setx0=off  InitialVoltage=0  Measurements=None
  Lm : spsSeriesRLCBranchLib/Series RLC Branch  LConnTagsString=__new0  RConnTagsString=__new0  BranchType=L  Resistance=88  Inductance=524.8e-6  SetiL0=off  InitialCurrent=0  Capacitance=2.62e-06  Setx0=off  InitialVoltage=0  Measurements=None
  Re : spsSeriesRLCBranchLib/Series RLC Branch  LConnTagsString=__new0  RConnTagsString=__new0  BranchType=R  Resistance=250  Inductance=6.3e-6  SetiL0=off  InitialCurrent=0  Capacitance=2.62e-06  Setx0=off  InitialVoltage=0  Measurements=None
  A : PMIOPort  Side=Left
  B : PMIOPort  Port=2  Side=Right
  connections:
  B/RConn1 -- Re/RConn1 -- Lm/RConn1 -- Cs/RConn1
  Lm/LConn1 -- Re/LConn1 -- LAir/RConn1
  LAir/LConn1 -- Cs/LConn1 -- A/RConn1

== system hcc_sm_v6_circuit2/Bridge2/Segment1/SaturableReactor ==
  note: C
  Cs : spsSeriesRLCBranchLib/Series RLC Branch  LConnTagsString=__new0  RConnTagsString=__new0  BranchType=C  Resistance=88  Inductance=6.3e-6  SetiL0=off  InitialCurrent=0  Capacitance=250e-12  Setx0=off  InitialVoltage=0  Measurements=None
  LAir : spsSeriesRLCBranchLib/Series RLC Branch  LConnTagsString=__new0  RConnTagsString=__new0  BranchType=L  Resistance=88  Inductance=6.3e-6  SetiL0=off  InitialCurrent=0  Capacitance=2.62e-06  Setx0=off  InitialVoltage=0  Measurements=None
  Lm : spsSeriesRLCBranchLib/Series RLC Branch  LConnTagsString=__new0  RConnTagsString=__new0  BranchType=L  Resistance=88  Inductance=524.8e-6  SetiL0=off  InitialCurrent=0  Capacitance=2.62e-06  Setx0=off  InitialVoltage=0  Measurements=None
  Re : spsSeriesRLCBranchLib/Series RLC Branch  LConnTagsString=__new0  RConnTagsString=__new0  BranchType=R  Resistance=250  Inductance=6.3e-6  SetiL0=off  InitialCurrent=0  Capacitance=2.62e-06  Setx0=off  InitialVoltage=0  Measurements=None
  A : PMIOPort  Side=Left
  B : PMIOPort  Port=2  Side=Right
  connections:
  B/RConn1 -- Re/RConn1 -- Lm/RConn1 -- Cs/RConn1
  Lm/LConn1 -- Re/LConn1 -- LAir/RConn1
  LAir/LConn1 -- Cs/LConn1 -- A/RConn1

== system hcc_sm_v6_circuit2/Bridge2/Segment2/SaturableReactor ==
  note: C
  Cs : spsSeriesRLCBranchLib/Series RLC Branch  LConnTagsString=__new0  RConnTagsString=__new0  BranchType=C  Resistance=88  Inductance=6.3e-6  SetiL0=off  InitialCurrent=0  Capacitance=250e-12  Setx0=off  InitialVoltage=0  Measurements=None
  LAir : spsSeriesRLCBranchLib/Series RLC Branch  LConnTagsString=__new0  RConnTagsString=__new0  BranchType=L  Resistance=88  Inductance=6.3e-6  SetiL0=off  InitialCurrent=0  Capacitance=2.62e-06  Setx0=off  InitialVoltage=0  Measurements=None
  Lm : spsSeriesRLCBranchLib/Series RLC Branch  LConnTagsString=__new0  RConnTagsString=__new0  BranchType=L  Resistance=88  Inductance=524.8e-6  SetiL0=off  InitialCurrent=0  Capacitance=2.62e-06  Setx0=off  InitialVoltage=0  Measurements=None
  Re : spsSeriesRLCBranchLib/Series RLC Branch  LConnTagsString=__new0  RConnTagsString=__new0  BranchType=R  Resistance=250  Inductance=6.3e-6  SetiL0=off  InitialCurrent=0  Capacitance=2.62e-06  Setx0=off  InitialVoltage=0  Measurements=None
  A : PMIOPort  Side=Left
  B : PMIOPort  Port=2  Side=Right
  connections:
  A/RConn1 -- Cs/LConn1 -- LAir/LConn1
  LAir/RConn1 -- Re/LConn1 -- Lm/LConn1
  Cs/RConn1 -- Lm/RConn1 -- Re/RConn1 -- B/RConn1

== system hcc_sm_v6_circuit2/Bridge2/Segment3/SaturableReactor ==
  note: C
  Cs : spsSeriesRLCBranchLib/Series RLC Branch  LConnTagsString=__new0  RConnTagsString=__new0  BranchType=C  Resistance=88  Inductance=6.3e-6  SetiL0=off  InitialCurrent=0  Capacitance=250e-12  Setx0=off  InitialVoltage=0  Measurements=None
  LAir : spsSeriesRLCBranchLib/Series RLC Branch  LConnTagsString=__new0  RConnTagsString=__new0  BranchType=L  Resistance=88  Inductance=6.3e-6  SetiL0=off  InitialCurrent=0  Capacitance=2.62e-06  Setx0=off  InitialVoltage=0  Measurements=None
  Lm : spsSeriesRLCBranchLib/Series RLC Branch  LConnTagsString=__new0  RConnTagsString=__new0  BranchType=L  Resistance=88  Inductance=524.8e-6  SetiL0=off  InitialCurrent=0  Capacitance=2.62e-06  Setx0=off  InitialVoltage=0  Measurements=None
  Re : spsSeriesRLCBranchLib/Series RLC Branch  LConnTagsString=__new0  RConnTagsString=__new0  BranchType=R  Resistance=250  Inductance=6.3e-6  SetiL0=off  InitialCurrent=0  Capacitance=2.62e-06  Setx0=off  InitialVoltage=0  Measurements=None
  A : PMIOPort  Side=Left
  B : PMIOPort  Port=2  Side=Right
  connections:
  B/RConn1 -- Re/RConn1 -- Lm/RConn1 -- Cs/RConn1
  Lm/LConn1 -- Re/LConn1 -- LAir/RConn1
  LAir/LConn1 -- Cs/LConn1 -- A/RConn1

== system hcc_sm_v6_circuit2/Bridge2/Segment4/SaturableReactor ==
  note: C
  Cs : spsSeriesRLCBranchLib/Series RLC Branch  LConnTagsString=__new0  RConnTagsString=__new0  BranchType=C  Resistance=88  Inductance=6.3e-6  SetiL0=off  InitialCurrent=0  Capacitance=250e-12  Setx0=off  InitialVoltage=0  Measurements=None
  LAir : spsSeriesRLCBranchLib/Series RLC Branch  LConnTagsString=__new0  RConnTagsString=__new0  BranchType=L  Resistance=88  Inductance=6.3e-6  SetiL0=off  InitialCurrent=0  Capacitance=2.62e-06  Setx0=off  InitialVoltage=0  Measurements=None
  Lm : spsSeriesRLCBranchLib/Series RLC Branch  LConnTagsString=__new0  RConnTagsString=__new0  BranchType=L  Resistance=88  Inductance=524.8e-6  SetiL0=off  InitialCurrent=0  Capacitance=2.62e-06  Setx0=off  InitialVoltage=0  Measurements=None
  Re : spsSeriesRLCBranchLib/Series RLC Branch  LConnTagsString=__new0  RConnTagsString=__new0  BranchType=R  Resistance=250  Inductance=6.3e-6  SetiL0=off  InitialCurrent=0  Capacitance=2.62e-06  Setx0=off  InitialVoltage=0  Measurements=None
  A : PMIOPort  Side=Left
  B : PMIOPort  Port=2  Side=Right
  connections:
  A/RConn1 -- Cs/LConn1 -- LAir/LConn1
  LAir/RConn1 -- Re/LConn1 -- Lm/LConn1
  Cs/RConn1 -- Lm/RConn1 -- Re/RConn1 -- B/RConn1

== system hcc_sm_v6_circuit2/Bridge3/Segment1/SaturableReactor ==
  note: C
  Cs : spsSeriesRLCBranchLib/Series RLC Branch  LConnTagsString=__new0  RConnTagsString=__new0  BranchType=C  Resistance=88  Inductance=6.3e-6  SetiL0=off  InitialCurrent=0  Capacitance=250e-12  Setx0=off  InitialVoltage=0  Measurements=None
  LAir : spsSeriesRLCBranchLib/Series RLC Branch  LConnTagsString=__new0  RConnTagsString=__new0  BranchType=L  Resistance=88  Inductance=6.3e-6  SetiL0=off  InitialCurrent=0  Capacitance=2.62e-06  Setx0=off  InitialVoltage=0  Measurements=None
  Lm : spsSeriesRLCBranchLib/Series RLC Branch  LConnTagsString=__new0  RConnTagsString=__new0  BranchType=L  Resistance=88  Inductance=524.8e-6  SetiL0=off  InitialCurrent=0  Capacitance=2.62e-06  Setx0=off  InitialVoltage=0  Measurements=None
  Re : spsSeriesRLCBranchLib/Series RLC Branch  LConnTagsString=__new0  RConnTagsString=__new0  BranchType=R  Resistance=250  Inductance=6.3e-6  SetiL0=off  InitialCurrent=0  Capacitance=2.62e-06  Setx0=off  InitialVoltage=0  Measurements=None
  A : PMIOPort  Side=Left
  B : PMIOPort  Port=2  Side=Right
  connections:
  A/RConn1 -- Cs/LConn1 -- LAir/LConn1
  LAir/RConn1 -- Re/LConn1 -- Lm/LConn1
  Cs/RConn1 -- Lm/RConn1 -- Re/RConn1 -- B/RConn1

== system hcc_sm_v6_circuit2/Bridge3/Segment2/SaturableReactor ==
  note: C
  Cs : spsSeriesRLCBranchLib/Series RLC Branch  LConnTagsString=__new0  RConnTagsString=__new0  BranchType=C  Resistance=88  Inductance=6.3e-6  SetiL0=off  InitialCurrent=0  Capacitance=250e-12  Setx0=off  InitialVoltage=0  Measurements=None
  LAir : spsSeriesRLCBranchLib/Series RLC Branch  LConnTagsString=__new0  RConnTagsString=__new0  BranchType=L  Resistance=88  Inductance=6.3e-6  SetiL0=off  InitialCurrent=0  Capacitance=2.62e-06  Setx0=off  InitialVoltage=0  Measurements=None
  Lm : spsSeriesRLCBranchLib/Series RLC Branch  LConnTagsString=__new0  RConnTagsString=__new0  BranchType=L  Resistance=88  Inductance=524.8e-6  SetiL0=off  InitialCurrent=0  Capacitance=2.62e-06  Setx0=off  InitialVoltage=0  Measurements=None
  Re : spsSeriesRLCBranchLib/Series RLC Branch  LConnTagsString=__new0  RConnTagsString=__new0  BranchType=R  Resistance=250  Inductance=6.3e-6  SetiL0=off  InitialCurrent=0  Capacitance=2.62e-06  Setx0=off  InitialVoltage=0  Measurements=None
  A : PMIOPort  Side=Left
  B : PMIOPort  Port=2  Side=Right
  connections:
  B/RConn1 -- Re/RConn1 -- Lm/RConn1 -- Cs/RConn1
  Lm/LConn1 -- Re/LConn1 -- LAir/RConn1
  LAir/LConn1 -- Cs/LConn1 -- A/RConn1

== system hcc_sm_v6_circuit2/Bridge3/Segment3/SaturableReactor ==
  note: C
  Cs : spsSeriesRLCBranchLib/Series RLC Branch  LConnTagsString=__new0  RConnTagsString=__new0  BranchType=C  Resistance=88  Inductance=6.3e-6  SetiL0=off  InitialCurrent=0  Capacitance=250e-12  Setx0=off  InitialVoltage=0  Measurements=None
  LAir : spsSeriesRLCBranchLib/Series RLC Branch  LConnTagsString=__new0  RConnTagsString=__new0  BranchType=L  Resistance=88  Inductance=6.3e-6  SetiL0=off  InitialCurrent=0  Capacitance=2.62e-06  Setx0=off  InitialVoltage=0  Measurements=None
  Lm : spsSeriesRLCBranchLib/Series RLC Branch  LConnTagsString=__new0  RConnTagsString=__new0  BranchType=L  Resistance=88  Inductance=524.8e-6  SetiL0=off  InitialCurrent=0  Capacitance=2.62e-06  Setx0=off  InitialVoltage=0  Measurements=None
  Re : spsSeriesRLCBranchLib/Series RLC Branch  LConnTagsString=__new0  RConnTagsString=__new0  BranchType=R  Resistance=250  Inductance=6.3e-6  SetiL0=off  InitialCurrent=0  Capacitance=2.62e-06  Setx0=off  InitialVoltage=0  Measurements=None
  A : PMIOPort  Side=Left
  B : PMIOPort  Port=2  Side=Right
  connections:
  A/RConn1 -- Cs/LConn1 -- LAir/LConn1
  LAir/RConn1 -- Re/LConn1 -- Lm/LConn1
  Cs/RConn1 -- Lm/RConn1 -- Re/RConn1 -- B/RConn1

== system hcc_sm_v6_circuit2/Bridge3/Segment4/SaturableReactor ==
  note: C
  Cs : spsSeriesRLCBranchLib/Series RLC Branch  LConnTagsString=__new0  RConnTagsString=__new0  BranchType=C  Resistance=88  Inductance=6.3e-6  SetiL0=off  InitialCurrent=0  Capacitance=250e-12  Setx0=off  InitialVoltage=0  Measurements=None
  LAir : spsSeriesRLCBranchLib/Series RLC Branch  LConnTagsString=__new0  RConnTagsString=__new0  BranchType=L  Resistance=88  Inductance=6.3e-6  SetiL0=off  InitialCurrent=0  Capacitance=2.62e-06  Setx0=off  InitialVoltage=0  Measurements=None
  Lm : spsSeriesRLCBranchLib/Series RLC Branch  LConnTagsString=__new0  RConnTagsString=__new0  BranchType=L  Resistance=88  Inductance=524.8e-6  SetiL0=off  InitialCurrent=0  Capacitance=2.62e-06  Setx0=off  InitialVoltage=0  Measurements=None
  Re : spsSeriesRLCBranchLib/Series RLC Branch  LConnTagsString=__new0  RConnTagsString=__new0  BranchType=R  Resistance=250  Inductance=6.3e-6  SetiL0=off  InitialCurrent=0  Capacitance=2.62e-06  Setx0=off  InitialVoltage=0  Measurements=None
  A : PMIOPort  Side=Left
  B : PMIOPort  Port=2  Side=Right
  connections:
  B/RConn1 -- Re/RConn1 -- Lm/RConn1 -- Cs/RConn1
  Lm/LConn1 -- Re/LConn1 -- LAir/RConn1
  LAir/LConn1 -- Cs/LConn1 -- A/RConn1

== system hcc_sm_v6_circuit2/Bridge4/Segment1/SaturableReactor ==
  note: C
  Cs : spsSeriesRLCBranchLib/Series RLC Branch  LConnTagsString=__new0  RConnTagsString=__new0  BranchType=C  Resistance=88  Inductance=6.3e-6  SetiL0=off  InitialCurrent=0  Capacitance=250e-12  Setx0=off  InitialVoltage=0  Measurements=None
  LAir : spsSeriesRLCBranchLib/Series RLC Branch  LConnTagsString=__new0  RConnTagsString=__new0  BranchType=L  Resistance=88  Inductance=6.3e-6  SetiL0=off  InitialCurrent=0  Capacitance=2.62e-06  Setx0=off  InitialVoltage=0  Measurements=None
  Lm : spsSeriesRLCBranchLib/Series RLC Branch  LConnTagsString=__new0  RConnTagsString=__new0  BranchType=L  Resistance=88  Inductance=524.8e-6  SetiL0=off  InitialCurrent=0  Capacitance=2.62e-06  Setx0=off  InitialVoltage=0  Measurements=None
  Re : spsSeriesRLCBranchLib/Series RLC Branch  LConnTagsString=__new0  RConnTagsString=__new0  BranchType=R  Resistance=250  Inductance=6.3e-6  SetiL0=off  InitialCurrent=0  Capacitance=2.62e-06  Setx0=off  InitialVoltage=0  Measurements=None
  A : PMIOPort  Side=Left
  B : PMIOPort  Port=2  Side=Right
  connections:
  B/RConn1 -- Re/RConn1 -- Lm/RConn1 -- Cs/RConn1
  Lm/LConn1 -- Re/LConn1 -- LAir/RConn1
  LAir/LConn1 -- Cs/LConn1 -- A/RConn1

== system hcc_sm_v6_circuit2/Bridge4/Segment2/SaturableReactor ==
  note: C
  Cs : spsSeriesRLCBranchLib/Series RLC Branch  LConnTagsString=__new0  RConnTagsString=__new0  BranchType=C  Resistance=88  Inductance=6.3e-6  SetiL0=off  InitialCurrent=0  Capacitance=250e-12  Setx0=off  InitialVoltage=0  Measurements=None
  LAir : spsSeriesRLCBranchLib/Series RLC Branch  LConnTagsString=__new0  RConnTagsString=__new0  BranchType=L  Resistance=88  Inductance=6.3e-6  SetiL0=off  InitialCurrent=0  Capacitance=2.62e-06  Setx0=off  InitialVoltage=0  Measurements=None
  Lm : spsSeriesRLCBranchLib/Series RLC Branch  LConnTagsString=__new0  RConnTagsString=__new0  BranchType=L  Resistance=88  Inductance=524.8e-6  SetiL0=off  InitialCurrent=0  Capacitance=2.62e-06  Setx0=off  InitialVoltage=0  Measurements=None
  Re : spsSeriesRLCBranchLib/Series RLC Branch  LConnTagsString=__new0  RConnTagsString=__new0  BranchType=R  Resistance=250  Inductance=6.3e-6  SetiL0=off  InitialCurrent=0  Capacitance=2.62e-06  Setx0=off  InitialVoltage=0  Measurements=None
  A : PMIOPort  Side=Left
  B : PMIOPort  Port=2  Side=Right
  connections:
  A/RConn1 -- Cs/LConn1 -- LAir/LConn1
  LAir/RConn1 -- Re/LConn1 -- Lm/LConn1
  Cs/RConn1 -- Lm/RConn1 -- Re/RConn1 -- B/RConn1

== system hcc_sm_v6_circuit2/Bridge4/Segment3/SaturableReactor ==
  note: C
  Cs : spsSeriesRLCBranchLib/Series RLC Branch  LConnTagsString=__new0  RConnTagsString=__new0  BranchType=C  Resistance=88  Inductance=6.3e-6  SetiL0=off  InitialCurrent=0  Capacitance=250e-12  Setx0=off  InitialVoltage=0  Measurements=None
  LAir : spsSeriesRLCBranchLib/Series RLC Branch  LConnTagsString=__new0  RConnTagsString=__new0  BranchType=L  Resistance=88  Inductance=6.3e-6  SetiL0=off  InitialCurrent=0  Capacitance=2.62e-06  Setx0=off  InitialVoltage=0  Measurements=None
  Lm : spsSeriesRLCBranchLib/Series RLC Branch  LConnTagsString=__new0  RConnTagsString=__new0  BranchType=L  Resistance=88  Inductance=524.8e-6  SetiL0=off  InitialCurrent=0  Capacitance=2.62e-06  Setx0=off  InitialVoltage=0  Measurements=None
  Re : spsSeriesRLCBranchLib/Series RLC Branch  LConnTagsString=__new0  RConnTagsString=__new0  BranchType=R  Resistance=250  Inductance=6.3e-6  SetiL0=off  InitialCurrent=0  Capacitance=2.62e-06  Setx0=off  InitialVoltage=0  Measurements=None
  A : PMIOPort  Side=Left
  B : PMIOPort  Port=2  Side=Right
  connections:
  B/RConn1 -- Re/RConn1 -- Lm/RConn1 -- Cs/RConn1
  Lm/LConn1 -- Re/LConn1 -- LAir/RConn1
  LAir/LConn1 -- Cs/LConn1 -- A/RConn1

== system hcc_sm_v6_circuit2/Bridge4/Segment4/SaturableReactor ==
  note: C
  Cs : spsSeriesRLCBranchLib/Series RLC Branch  LConnTagsString=__new0  RConnTagsString=__new0  BranchType=C  Resistance=88  Inductance=6.3e-6  SetiL0=off  InitialCurrent=0  Capacitance=250e-12  Setx0=off  InitialVoltage=0  Measurements=None
  LAir : spsSeriesRLCBranchLib/Series RLC Branch  LConnTagsString=__new0  RConnTagsString=__new0  BranchType=L  Resistance=88  Inductance=6.3e-6  SetiL0=off  InitialCurrent=0  Capacitance=2.62e-06  Setx0=off  InitialVoltage=0  Measurements=None
  Lm : spsSeriesRLCBranchLib/Series RLC Branch  LConnTagsString=__new0  RConnTagsString=__new0  BranchType=L  Resistance=88  Inductance=524.8e-6  SetiL0=off  InitialCurrent=0  Capacitance=2.62e-06  Setx0=off  InitialVoltage=0  Measurements=None
  Re : spsSeriesRLCBranchLib/Series RLC Branch  LConnTagsString=__new0  RConnTagsString=__new0  BranchType=R  Resistance=250  Inductance=6.3e-6  SetiL0=off  InitialCurrent=0  Capacitance=2.62e-06  Setx0=off  InitialVoltage=0  Measurements=None
  A : PMIOPort  Side=Left
  B : PMIOPort  Port=2  Side=Right
  connections:
  A/RConn1 -- Cs/LConn1 -- LAir/LConn1
  LAir/RConn1 -- Re/LConn1 -- Lm/LConn1
  Cs/RConn1 -- Lm/RConn1 -- Re/RConn1 -- B/RConn1

== system hcc_sm_v6_circuit2/Bridge5/Segment1/SaturableReactor ==
  note: C
  Cs : spsSeriesRLCBranchLib/Series RLC Branch  LConnTagsString=__new0  RConnTagsString=__new0  BranchType=C  Resistance=88  Inductance=6.3e-6  SetiL0=off  InitialCurrent=0  Capacitance=250e-12  Setx0=off  InitialVoltage=0  Measurements=None
  LAir : spsSeriesRLCBranchLib/Series RLC Branch  LConnTagsString=__new0  RConnTagsString=__new0  BranchType=L  Resistance=88  Inductance=6.3e-6  SetiL0=off  InitialCurrent=0  Capacitance=2.62e-06  Setx0=off  InitialVoltage=0  Measurements=None
  Lm : spsSeriesRLCBranchLib/Series RLC Branch  LConnTagsString=__new0  RConnTagsString=__new0  BranchType=L  Resistance=88  Inductance=524.8e-6  SetiL0=off  InitialCurrent=0  Capacitance=2.62e-06  Setx0=off  InitialVoltage=0  Measurements=None
  Re : spsSeriesRLCBranchLib/Series RLC Branch  LConnTagsString=__new0  RConnTagsString=__new0  BranchType=R  Resistance=250  Inductance=6.3e-6  SetiL0=off  InitialCurrent=0  Capacitance=2.62e-06  Setx0=off  InitialVoltage=0  Measurements=None
  A : PMIOPort  Side=Left
  B : PMIOPort  Port=2  Side=Right
  connections:
  A/RConn1 -- Cs/LConn1 -- LAir/LConn1
  LAir/RConn1 -- Re/LConn1 -- Lm/LConn1
  Cs/RConn1 -- Lm/RConn1 -- Re/RConn1 -- B/RConn1

== system hcc_sm_v6_circuit2/Bridge5/Segment2/SaturableReactor ==
  note: C
  Cs : spsSeriesRLCBranchLib/Series RLC Branch  LConnTagsString=__new0  RConnTagsString=__new0  BranchType=C  Resistance=88  Inductance=6.3e-6  SetiL0=off  InitialCurrent=0  Capacitance=250e-12  Setx0=off  InitialVoltage=0  Measurements=None
  LAir : spsSeriesRLCBranchLib/Series RLC Branch  LConnTagsString=__new0  RConnTagsString=__new0  BranchType=L  Resistance=88  Inductance=6.3e-6  SetiL0=off  InitialCurrent=0  Capacitance=2.62e-06  Setx0=off  InitialVoltage=0  Measurements=None
  Lm : spsSeriesRLCBranchLib/Series RLC Branch  LConnTagsString=__new0  RConnTagsString=__new0  BranchType=L  Resistance=88  Inductance=524.8e-6  SetiL0=off  InitialCurrent=0  Capacitance=2.62e-06  Setx0=off  InitialVoltage=0  Measurements=None
  Re : spsSeriesRLCBranchLib/Series RLC Branch  LConnTagsString=__new0  RConnTagsString=__new0  BranchType=R  Resistance=250  Inductance=6.3e-6  SetiL0=off  InitialCurrent=0  Capacitance=2.62e-06  Setx0=off  InitialVoltage=0  Measurements=None
  A : PMIOPort  Side=Left
  B : PMIOPort  Port=2  Side=Right
  connections:
  B/RConn1 -- Re/RConn1 -- Lm/RConn1 -- Cs/RConn1
  Lm/LConn1 -- Re/LConn1 -- LAir/RConn1
  LAir/LConn1 -- Cs/LConn1 -- A/RConn1

== system hcc_sm_v6_circuit2/Bridge5/Segment3/SaturableReactor ==
  note: C
  Cs : spsSeriesRLCBranchLib/Series RLC Branch  LConnTagsString=__new0  RConnTagsString=__new0  BranchType=C  Resistance=88  Inductance=6.3e-6  SetiL0=off  InitialCurrent=0  Capacitance=250e-12  Setx0=off  InitialVoltage=0  Measurements=None
  LAir : spsSeriesRLCBranchLib/Series RLC Branch  LConnTagsString=__new0  RConnTagsString=__new0  BranchType=L  Resistance=88  Inductance=6.3e-6  SetiL0=off  InitialCurrent=0  Capacitance=2.62e-06  Setx0=off  InitialVoltage=0  Measurements=None
  Lm : spsSeriesRLCBranchLib/Series RLC Branch  LConnTagsString=__new0  RConnTagsString=__new0  BranchType=L  Resistance=88  Inductance=524.8e-6  SetiL0=off  InitialCurrent=0  Capacitance=2.62e-06  Setx0=off  InitialVoltage=0  Measurements=None
  Re : spsSeriesRLCBranchLib/Series RLC Branch  LConnTagsString=__new0  RConnTagsString=__new0  BranchType=R  Resistance=250  Inductance=6.3e-6  SetiL0=off  InitialCurrent=0  Capacitance=2.62e-06  Setx0=off  InitialVoltage=0  Measurements=None
  A : PMIOPort  Side=Left
  B : PMIOPort  Port=2  Side=Right
  connections:
  A/RConn1 -- Cs/LConn1 -- LAir/LConn1
  LAir/RConn1 -- Re/LConn1 -- Lm/LConn1
  Cs/RConn1 -- Lm/RConn1 -- Re/RConn1 -- B/RConn1
